simulink model "junyakaiguangai5"  (Simulink 8.8)
settings: Solver=ode4  StartTime=0.0  StopTime=inf  FixedStep=0.001  RelTol=1e-3  EnableMultiTasking=on
undefined symbols (not defined in the file or in its folder): mdaadlink6208, sigbuilder_block
libraries: xpcobsoletelib x24, slrtlib x2, simulink x1
(part 2 of 3)

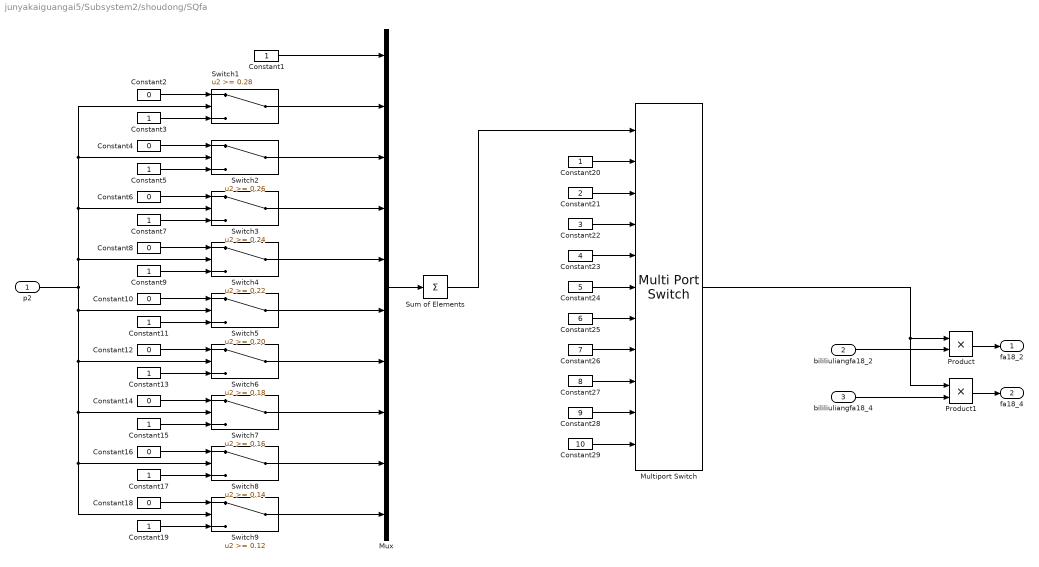
== system junyakaiguangai5/Subsystem2/shoudong/SQfa ==
  p2 : Inport
  bililiuliangfa18_2 : Inport  Port=2
  bililiuliangfa18_4 : Inport  Port=3
  Constant{1,3,5,7,9,11,13,15,17,19..20} (11 alike) : Constant
  Constant{2,4,6,8,10,12,14,16,18} (9 alike) : Constant  Value=0
  Constant21 : Constant  Value=2
  Constant22 : Constant  Value=3
  Constant23 : Constant  Value=4
  Constant24 : Constant  Value=5
  Constant25 : Constant  Value=6
  Constant26 : Constant  Value=7
  Constant27 : Constant  Value=8
  Constant28 : Constant  Value=9
  Constant29 : Constant  Value=10
  Multiport Switch : MultiPortSwitch  Inputs=10
  Mux : Mux  Inputs=10
  Product : Product  RndMeth=Zero
  Product1 : Product  RndMeth=Zero
  Sum of Elements : Sum  Inputs=+
  Switch1 : Switch  Threshold=0.28
  Switch2 : Switch  Threshold=0.26
  Switch3 : Switch  Threshold=0.24
  Switch4 : Switch  Threshold=0.22
  Switch5 : Switch  Threshold=0.20
  Switch6 : Switch  Threshold=0.18
  Switch7 : Switch  Threshold=0.16
  Switch8 : Switch  Threshold=0.14
  Switch9 : Switch  Threshold=0.12
  fa18_2 : Outport
  fa18_4 : Outport  Port=2
  wires:
  Constant2/1 -> Switch1/1
  Constant3/1 -> Switch1/3
  Constant4/1 -> Switch2/1
  Constant5/1 -> Switch2/3
  Constant6/1 -> Switch3/1
  Constant7/1 -> Switch3/3
  Constant8/1 -> Switch4/1
  Constant9/1 -> Switch4/3
  Constant10/1 -> Switch5/1
  Constant11/1 -> Switch5/3
  Constant12/1 -> Switch6/1
  Constant13/1 -> Switch6/3
  Constant14/1 -> Switch7/1
  Constant15/1 -> Switch7/3
  p2/1 -> Switch1/2, Switch2/2, Switch3/2, Switch4/2, Switch6/2, Switch7/2, Switch8/2, Switch9/2, Switch5/2
  Mux/1 -> Sum of Elements/1
  Sum of Elements/1 -> Multiport Switch/1
  Constant1/1 -> Mux/1
  Switch1/1 -> Mux/2
  Switch2/1 -> Mux/3
  Switch3/1 -> Mux/4
  Switch4/1 -> Mux/5
  Switch5/1 -> Mux/6
  Switch6/1 -> Mux/7
  Switch7/1 -> Mux/8
  Switch8/1 -> Mux/9
  Switch9/1 -> Mux/10
  Constant16/1 -> Switch8/1
  Constant17/1 -> Switch8/3
  Constant18/1 -> Switch9/1
  Constant19/1 -> Switch9/3
  Multiport Switch/1 -> Product/1, Product1/1
  Constant20/1 -> Multiport Switch/2
  Constant21/1 -> Multiport Switch/3
  Constant22/1 -> Multiport Switch/4
  Constant23/1 -> Multiport Switch/5
  Constant24/1 -> Multiport Switch/6
  Constant25/1 -> Multiport Switch/7
  Constant26/1 -> Multiport Switch/8
  Constant27/1 -> Multiport Switch/9
  Constant28/1 -> Multiport Switch/10
  Constant29/1 -> Multiport Switch/11
  bililiuliangfa18_2/1 -> Product/2
  bililiuliangfa18_4/1 -> Product1/2
  Product/1 -> fa18_2/1
  Product1/1 -> fa18_4/1

== system junyakaiguangai5/Subsystem2/shoudong/Subsystem1 ==
  kaigaikaishi : Inport
  guangaikaishi : Inport  Port=2
  xkgg : Inport  Port=3
  Add1 : Sum
  Constant : Constant  Value=2
  Constant1 : Constant  Value=0
  Gain : Gain
  Gain1 : Gain
  Multiport Switch : MultiPortSwitch
  Product : Product
  Signal Builder : Subsystem  Tag=STV Subsys  LoadFcn=sigbuilder_block('load');  StartFcn=sigbuilder_block('start');  StopFcn=sigbuilder_block('stop');  ClipboardFcn=sigbuilder_block('clipboard');  mask(Sigbuilder block){tuvar=[0:10]}
      mask help: Simulink:masks:SigbuilderBlock_MD
      mask init:
      | if ~strcmp(get_param(bdroot(gcbh),'SimulationStatus'),'stopped') tuvar = sigbuilder_block('maskInit'); end
      settings: CopyFcn=sigbuilder_block('copy');  DeleteFcn=sigbuilder_block('delete');  ModelCloseFcn=sigbuilder_block('modelClose');  PreSaveFcn=sigbuilder_block('preSave');  PauseFcn=sigbuilder_block('pause');  ContinueFcn=sigbuilder_block('continue');  NameChangeFcn=sigbuilder_block('namechange');  OpenFcn=sigbuilder_block('open',[437.6 199.2 550.4 400 ]);  CloseFcn=sigbuilder_block('close');
      mask Display: plot(0, 0, 100, 100,[2, 2, 32, 32, 2], [68, 8, 8, 68, 68],[32, 2], [38, 38], [32, 19, 2],[53, 60, 44], [32, 17, 17, 2],[16, 16, 31, 31]);txt = getActiveGroup(gcbh);text(2, 100, txt,'verticalAlignment', 'top');
  Signal Builder1 : Subsystem  Tag=STV Subsys  LoadFcn=sigbuilder_block('load');  StartFcn=sigbuilder_block('start');  StopFcn=sigbuilder_block('stop');  ClipboardFcn=sigbuilder_block('clipboard');  mask(Sigbuilder block){tuvar=[0:10]}
      mask help: Simulink:masks:SigbuilderBlock_MD
      mask init:
      | if ~strcmp(get_param(bdroot(gcbh),'SimulationStatus'),'stopped') tuvar = sigbuilder_block('maskInit'); end
      settings: CopyFcn=sigbuilder_block('copy');  DeleteFcn=sigbuilder_block('delete');  ModelCloseFcn=sigbuilder_block('modelClose');  PreSaveFcn=sigbuilder_block('preSave');  PauseFcn=sigbuilder_block('pause');  ContinueFcn=sigbuilder_block('continue');  NameChangeFcn=sigbuilder_block('namechange');  OpenFcn=sigbuilder_block('open',[437.6 199.2 550.4 400 ]);  CloseFcn=sigbuilder_block('close');
      mask Display: plot(0, 0, 100, 100,[2, 2, 32, 32, 2], [68, 8, 8, 68, 68],[32, 2], [38, 38], [32, 19, 2],[53, 60, 44], [32, 17, 17, 2],[16, 16, 31, 31]);txt = getActiveGroup(gcbh);text(2, 100, txt,'verticalAlignment', 'top');
  Sum : Sum  Inputs=|+-
  Sum1 : Sum  Inputs=|+-
  Out1 : Outport
  wires:
  guangaikaishi/1 -> Product/1
  Constant/1 -> Product/2
  kaigaikaishi/1 -> Add1/1
  Product/1 -> Add1/2
  Add1/1 -> Multiport Switch/1
  Multiport Switch/1 -> Out1/1
  Signal Builder/1(Signal 1) -> Sum/1
  xkgg/1 -> Sum1/2, Sum/2
  Sum/1 -> Gain/1
  Gain/1 -> Multiport Switch/2
  Signal Builder1/1(Signal 1) -> Sum1/1
  Sum1/1 -> Gain1/1
  Gain1/1 -> Multiport Switch/3
  Constant1/1 -> Multiport Switch/4

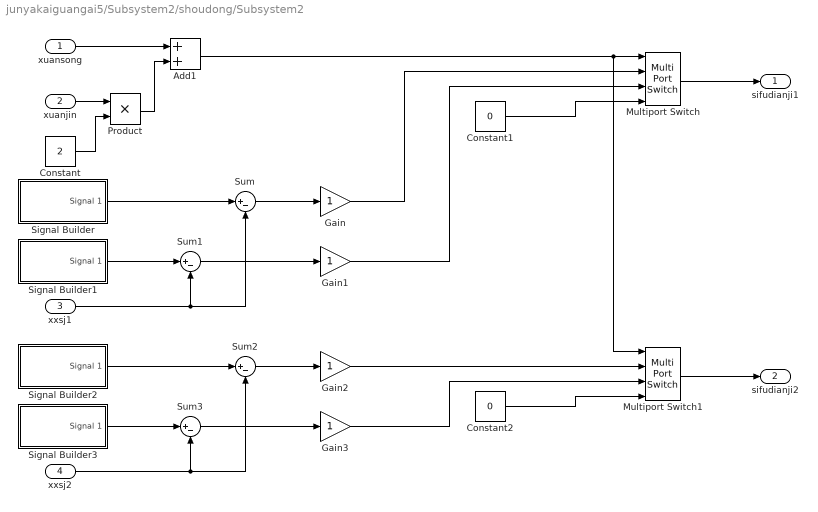
== system junyakaiguangai5/Subsystem2/shoudong/Subsystem2 ==
  xuansong : Inport
  xuanjin : Inport  Port=2
  xxsj1 : Inport  Port=3
  xxsj2 : Inport  Port=4
  Add1 : Sum
  Constant : Constant  Value=2
  Constant1 : Constant  Value=0
  Constant2 : Constant  Value=0
  Gain{,1..3} (4 alike) : Gain
  Multiport Switch : MultiPortSwitch
  Multiport Switch1 : MultiPortSwitch
  Product : Product
  Signal Builder : Subsystem  Tag=STV Subsys  LoadFcn=sigbuilder_block('load');  StartFcn=sigbuilder_block('start');  StopFcn=sigbuilder_block('stop');  ClipboardFcn=sigbuilder_block('clipboard');  mask(Sigbuilder block){tuvar=[0:10]}
      mask help: Simulink:masks:SigbuilderBlock_MD
      mask init:
      | if ~strcmp(get_param(bdroot(gcbh),'SimulationStatus'),'stopped') tuvar = sigbuilder_block('maskInit'); end
      settings: CopyFcn=sigbuilder_block('copy');  DeleteFcn=sigbuilder_block('delete');  ModelCloseFcn=sigbuilder_block('modelClose');  PreSaveFcn=sigbuilder_block('preSave');  PauseFcn=sigbuilder_block('pause');  ContinueFcn=sigbuilder_block('continue');  NameChangeFcn=sigbuilder_block('namechange');  OpenFcn=sigbuilder_block('open',[437.6 199.2 550.4 400 ]);  CloseFcn=sigbuilder_block('close');
      mask Display: plot(0, 0, 100, 100,[2, 2, 32, 32, 2], [68, 8, 8, 68, 68],[32, 2], [38, 38], [32, 19, 2],[53, 60, 44], [32, 17, 17, 2],[16, 16, 31, 31]);txt = getActiveGroup(gcbh);text(2, 100, txt,'verticalAlignment', 'top');
  Signal Builder1 : Subsystem  Tag=STV Subsys  LoadFcn=sigbuilder_block('load');  StartFcn=sigbuilder_block('start');  StopFcn=sigbuilder_block('stop');  ClipboardFcn=sigbuilder_block('clipboard');  mask(Sigbuilder block){tuvar=[0:10]}
      mask help: Simulink:masks:SigbuilderBlock_MD
      mask init:
      | if ~strcmp(get_param(bdroot(gcbh),'SimulationStatus'),'stopped') tuvar = sigbuilder_block('maskInit'); end
      settings: CopyFcn=sigbuilder_block('copy');  DeleteFcn=sigbuilder_block('delete');  ModelCloseFcn=sigbuilder_block('modelClose');  PreSaveFcn=sigbuilder_block('preSave');  PauseFcn=sigbuilder_block('pause');  ContinueFcn=sigbuilder_block('continue');  NameChangeFcn=sigbuilder_block('namechange');  OpenFcn=sigbuilder_block('open',[437.6 199.2 550.4 400 ]);  CloseFcn=sigbuilder_block('close');
      mask Display: plot(0, 0, 100, 100,[2, 2, 32, 32, 2], [68, 8, 8, 68, 68],[32, 2], [38, 38], [32, 19, 2],[53, 60, 44], [32, 17, 17, 2],[16, 16, 31, 31]);txt = getActiveGroup(gcbh);text(2, 100, txt,'verticalAlignment', 'top');
  Signal Builder2 : Subsystem  Tag=STV Subsys  LoadFcn=sigbuilder_block('load');  StartFcn=sigbuilder_block('start');  StopFcn=sigbuilder_block('stop');  ClipboardFcn=sigbuilder_block('clipboard');  mask(Sigbuilder block){tuvar=[0:10]}
      mask help: Simulink:masks:SigbuilderBlock_MD
      mask init:
      | if ~strcmp(get_param(bdroot(gcbh),'SimulationStatus'),'stopped') tuvar = sigbuilder_block('maskInit'); end
      settings: CopyFcn=sigbuilder_block('copy');  DeleteFcn=sigbuilder_block('delete');  ModelCloseFcn=sigbuilder_block('modelClose');  PreSaveFcn=sigbuilder_block('preSave');  PauseFcn=sigbuilder_block('pause');  ContinueFcn=sigbuilder_block('continue');  NameChangeFcn=sigbuilder_block('namechange');  OpenFcn=sigbuilder_block('open',[437.6 199.2 550.4 400 ]);  CloseFcn=sigbuilder_block('close');
      mask Display: plot(0, 0, 100, 100,[2, 2, 32, 32, 2], [68, 8, 8, 68, 68],[32, 2], [38, 38], [32, 19, 2],[53, 60, 44], [32, 17, 17, 2],[16, 16, 31, 31]);txt = getActiveGroup(gcbh);text(2, 100, txt,'verticalAlignment', 'top');
  Signal Builder3 : Subsystem  Tag=STV Subsys  LoadFcn=sigbuilder_block('load');  StartFcn=sigbuilder_block('start');  StopFcn=sigbuilder_block('stop');  ClipboardFcn=sigbuilder_block('clipboard');  mask(Sigbuilder block){tuvar=[0:10]}
      mask help: Simulink:masks:SigbuilderBlock_MD
      mask init:
      | if ~strcmp(get_param(bdroot(gcbh),'SimulationStatus'),'stopped') tuvar = sigbuilder_block('maskInit'); end
      settings: CopyFcn=sigbuilder_block('copy');  DeleteFcn=sigbuilder_block('delete');  ModelCloseFcn=sigbuilder_block('modelClose');  PreSaveFcn=sigbuilder_block('preSave');  PauseFcn=sigbuilder_block('pause');  ContinueFcn=sigbuilder_block('continue');  NameChangeFcn=sigbuilder_block('namechange');  OpenFcn=sigbuilder_block('open',[437.6 199.2 550.4 400 ]);  CloseFcn=sigbuilder_block('close');
      mask Display: plot(0, 0, 100, 100,[2, 2, 32, 32, 2], [68, 8, 8, 68, 68],[32, 2], [38, 38], [32, 19, 2],[53, 60, 44], [32, 17, 17, 2],[16, 16, 31, 31]);txt = getActiveGroup(gcbh);text(2, 100, txt,'verticalAlignment', 'top');
  Sum{,1..3} (4 alike) : Sum  Inputs=|+-
  sifudianji1 : Outport
  sifudianji2 : Outport  Port=2
  wires:
  Constant1/1 -> Multiport Switch/4
  Gain1/1 -> Multiport Switch/3
  Sum1/1 -> Gain1/1
  Signal Builder1/1(Signal 1) -> Sum1/1
  Gain/1 -> Multiport Switch/2
  Sum/1 -> Gain/1
  xxsj1/1 -> Sum/2, Sum1/2
  Signal Builder/1(Signal 1) -> Sum/1
  Multiport Switch/1 -> sifudianji1/1
  Add1/1 -> Multiport Switch1/1, Multiport Switch/1
  Product/1 -> Add1/2
  xuansong/1 -> Add1/1
  Constant/1 -> Product/2
  xuanjin/1 -> Product/1
  Multiport Switch1/1 -> sifudianji2/1
  Signal Builder2/1(Signal 1) -> Sum2/1
  xxsj2/1 -> Sum2/2, Sum3/2
  Sum2/1 -> Gain2/1
  Gain2/1 -> Multiport Switch1/2
  Signal Builder3/1(Signal 1) -> Sum3/1
  Sum3/1 -> Gain3/1
  Gain3/1 -> Multiport Switch1/3
  Constant2/1 -> Multiport Switch1/4

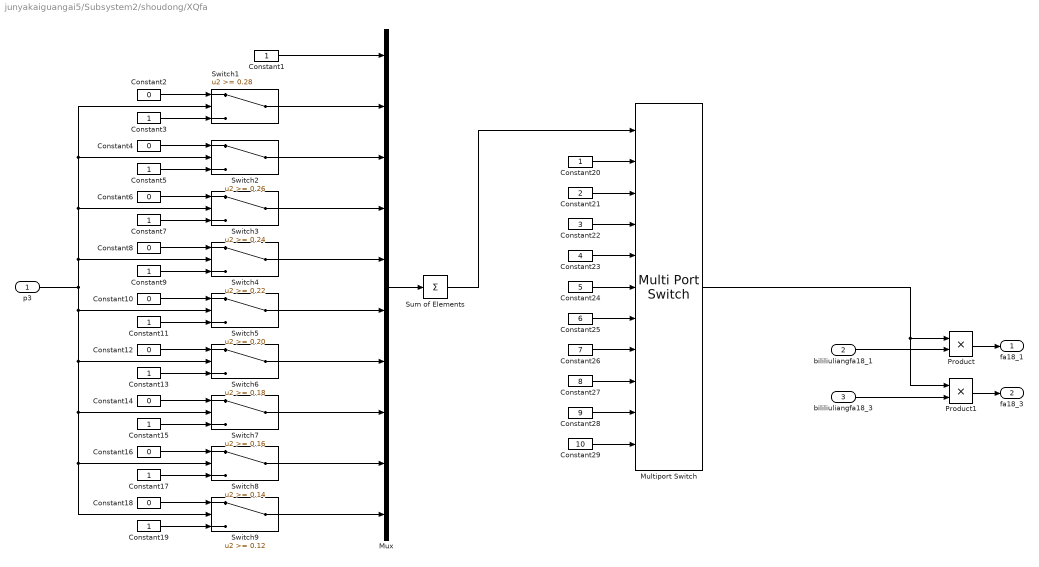
== system junyakaiguangai5/Subsystem2/shoudong/XQfa ==
  p3 : Inport
  bililiuliangfa18_1 : Inport  Port=2
  bililiuliangfa18_3 : Inport  Port=3
  Constant{1,3,5,7,9,11,13,15,17,19..20} (11 alike) : Constant
  Constant{2,4,6,8,10,12,14,16,18} (9 alike) : Constant  Value=0
  Constant21 : Constant  Value=2
  Constant22 : Constant  Value=3
  Constant23 : Constant  Value=4
  Constant24 : Constant  Value=5
  Constant25 : Constant  Value=6
  Constant26 : Constant  Value=7
  Constant27 : Constant  Value=8
  Constant28 : Constant  Value=9
  Constant29 : Constant  Value=10
  Multiport Switch : MultiPortSwitch  Inputs=10
  Mux : Mux  Inputs=10
  Product : Product  RndMeth=Zero
  Product1 : Product  RndMeth=Zero
  Sum of Elements : Sum  Inputs=+
  Switch1 : Switch  Threshold=0.28
  Switch2 : Switch  Threshold=0.26
  Switch3 : Switch  Threshold=0.24
  Switch4 : Switch  Threshold=0.22
  Switch5 : Switch  Threshold=0.20
  Switch6 : Switch  Threshold=0.18
  Switch7 : Switch  Threshold=0.16
  Switch8 : Switch  Threshold=0.14
  Switch9 : Switch  Threshold=0.12
  fa18_1 : Outport
  fa18_3 : Outport  Port=2
  wires:
  Product1/1 -> fa18_3/1
  Product/1 -> fa18_1/1
  bililiuliangfa18_3/1 -> Product1/2
  bililiuliangfa18_1/1 -> Product/2
  Constant29/1 -> Multiport Switch/11
  Constant28/1 -> Multiport Switch/10
  Constant27/1 -> Multiport Switch/9
  Constant26/1 -> Multiport Switch/8
  Constant25/1 -> Multiport Switch/7
  Constant24/1 -> Multiport Switch/6
  Constant23/1 -> Multiport Switch/5
  Constant22/1 -> Multiport Switch/4
  Constant21/1 -> Multiport Switch/3
  Constant20/1 -> Multiport Switch/2
  Multiport Switch/1 -> Product1/1, Product/1
  Constant19/1 -> Switch9/3
  Constant18/1 -> Switch9/1
  Constant17/1 -> Switch8/3
  Constant16/1 -> Switch8/1
  Switch9/1 -> Mux/10
  Switch8/1 -> Mux/9
  Switch7/1 -> Mux/8
  Switch6/1 -> Mux/7
  Switch5/1 -> Mux/6
  Switch4/1 -> Mux/5
  Switch3/1 -> Mux/4
  Switch2/1 -> Mux/3
  Switch1/1 -> Mux/2
  Constant1/1 -> Mux/1
  Sum of Elements/1 -> Multiport Switch/1
  Mux/1 -> Sum of Elements/1
  p3/1 -> Switch5/2, Switch9/2, Switch8/2, Switch7/2, Switch6/2, Switch4/2, Switch3/2, Switch2/2, Switch1/2
  Constant15/1 -> Switch7/3
  Constant14/1 -> Switch7/1
  Constant13/1 -> Switch6/3
  Constant12/1 -> Switch6/1
  Constant11/1 -> Switch5/3
  Constant10/1 -> Switch5/1
  Constant9/1 -> Switch4/3
  Constant8/1 -> Switch4/1
  Constant7/1 -> Switch3/3
  Constant6/1 -> Switch3/1
  Constant5/1 -> Switch2/3
  Constant4/1 -> Switch2/1
  Constant3/1 -> Switch1/3
  Constant2/1 -> Switch1/1

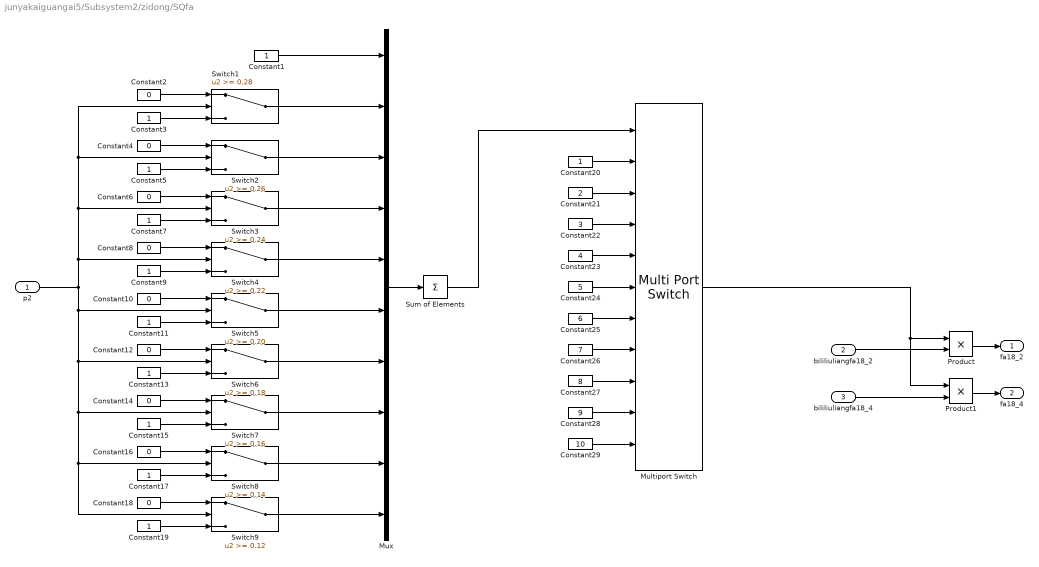
== system junyakaiguangai5/Subsystem2/zidong/SQfa ==
  p2 : Inport
  bililiuliangfa18_2 : Inport  Port=2
  bililiuliangfa18_4 : Inport  Port=3
  Constant{1,3,5,7,9,11,13,15,17,19..20} (11 alike) : Constant
  Constant{2,4,6,8,10,12,14,16,18} (9 alike) : Constant  Value=0
  Constant21 : Constant  Value=2
  Constant22 : Constant  Value=3
  Constant23 : Constant  Value=4
  Constant24 : Constant  Value=5
  Constant25 : Constant  Value=6
  Constant26 : Constant  Value=7
  Constant27 : Constant  Value=8
  Constant28 : Constant  Value=9
  Constant29 : Constant  Value=10
  Multiport Switch : MultiPortSwitch  Inputs=10
  Mux : Mux  Inputs=10
  Product : Product  RndMeth=Zero
  Product1 : Product  RndMeth=Zero
  Sum of Elements : Sum  Inputs=+
  Switch1 : Switch  Threshold=0.28
  Switch2 : Switch  Threshold=0.26
  Switch3 : Switch  Threshold=0.24
  Switch4 : Switch  Threshold=0.22
  Switch5 : Switch  Threshold=0.20
  Switch6 : Switch  Threshold=0.18
  Switch7 : Switch  Threshold=0.16
  Switch8 : Switch  Threshold=0.14
  Switch9 : Switch  Threshold=0.12
  fa18_2 : Outport
  fa18_4 : Outport  Port=2
  wires:
  Product1/1 -> fa18_4/1
  Product/1 -> fa18_2/1
  bililiuliangfa18_4/1 -> Product1/2
  bililiuliangfa18_2/1 -> Product/2
  Constant29/1 -> Multiport Switch/11
  Constant28/1 -> Multiport Switch/10
  Constant27/1 -> Multiport Switch/9
  Constant26/1 -> Multiport Switch/8
  Constant25/1 -> Multiport Switch/7
  Constant24/1 -> Multiport Switch/6
  Constant23/1 -> Multiport Switch/5
  Constant22/1 -> Multiport Switch/4
  Constant21/1 -> Multiport Switch/3
  Constant20/1 -> Multiport Switch/2
  Multiport Switch/1 -> Product1/1, Product/1
  Constant19/1 -> Switch9/3
  Constant18/1 -> Switch9/1
  Constant17/1 -> Switch8/3
  Constant16/1 -> Switch8/1
  Switch9/1 -> Mux/10
  Switch8/1 -> Mux/9
  Switch7/1 -> Mux/8
  Switch6/1 -> Mux/7
  Switch5/1 -> Mux/6
  Switch4/1 -> Mux/5
  Switch3/1 -> Mux/4
  Switch2/1 -> Mux/3
  Switch1/1 -> Mux/2
  Constant1/1 -> Mux/1
  Sum of Elements/1 -> Multiport Switch/1
  Mux/1 -> Sum of Elements/1
  p2/1 -> Switch5/2, Switch9/2, Switch8/2, Switch7/2, Switch6/2, Switch4/2, Switch3/2, Switch2/2, Switch1/2
  Constant15/1 -> Switch7/3
  Constant14/1 -> Switch7/1
  Constant13/1 -> Switch6/3
  Constant12/1 -> Switch6/1
  Constant11/1 -> Switch5/3
  Constant10/1 -> Switch5/1
  Constant9/1 -> Switch4/3
  Constant8/1 -> Switch4/1
  Constant7/1 -> Switch3/3
  Constant6/1 -> Switch3/1
  Constant5/1 -> Switch2/3
  Constant4/1 -> Switch2/1
  Constant3/1 -> Switch1/3
  Constant2/1 -> Switch1/1

== system junyakaiguangai5/Subsystem2/zidong/Subsystem ==
  kaigaikaishi : Inport
  guangaikaishi : Inport  Port=2
  xkgg : Inport  Port=3
  Add1 : Sum
  Constant : Constant  Value=2
  Constant1 : Constant  Value=0
  Gain : Gain
  Gain1 : Gain
  Multiport Switch : MultiPortSwitch
  Product : Product
  Signal Builder : Subsystem  Tag=STV Subsys  LoadFcn=sigbuilder_block('load');  StartFcn=sigbuilder_block('start');  StopFcn=sigbuilder_block('stop');  ClipboardFcn=sigbuilder_block('clipboard');  mask(Sigbuilder block){tuvar=[0:10]}
      mask help: Simulink:masks:SigbuilderBlock_MD
      mask init:
      | if ~strcmp(get_param(bdroot(gcbh),'SimulationStatus'),'stopped') tuvar = sigbuilder_block('maskInit'); end
      settings: CopyFcn=sigbuilder_block('copy');  DeleteFcn=sigbuilder_block('delete');  ModelCloseFcn=sigbuilder_block('modelClose');  PreSaveFcn=sigbuilder_block('preSave');  PauseFcn=sigbuilder_block('pause');  ContinueFcn=sigbuilder_block('continue');  NameChangeFcn=sigbuilder_block('namechange');  OpenFcn=sigbuilder_block('open',[440.25 156.75 544.5 354.75 ]);  CloseFcn=sigbuilder_block('close');
      mask Display: plot(0, 0, 100, 100,[2, 2, 32, 32, 2], [68, 8, 8, 68, 68],[32, 2], [38, 38], [32, 19, 2],[53, 60, 44], [32, 17, 17, 2],[16, 16, 31, 31]);txt = getActiveGroup(gcbh);text(2, 100, txt,'verticalAlignment', 'top');
  Signal Builder1 : Subsystem  Tag=STV Subsys  LoadFcn=sigbuilder_block('load');  StartFcn=sigbuilder_block('start');  StopFcn=sigbuilder_block('stop');  ClipboardFcn=sigbuilder_block('clipboard');  mask(Sigbuilder block){tuvar=[0:10]}
      mask help: Simulink:masks:SigbuilderBlock_MD
      mask init:
      | if ~strcmp(get_param(bdroot(gcbh),'SimulationStatus'),'stopped') tuvar = sigbuilder_block('maskInit'); end
      settings: CopyFcn=sigbuilder_block('copy');  DeleteFcn=sigbuilder_block('delete');  ModelCloseFcn=sigbuilder_block('modelClose');  PreSaveFcn=sigbuilder_block('preSave');  PauseFcn=sigbuilder_block('pause');  ContinueFcn=sigbuilder_block('continue');  NameChangeFcn=sigbuilder_block('namechange');  OpenFcn=sigbuilder_block('open',[437.6 199.2 550.4 400 ]);  CloseFcn=sigbuilder_block('close');
      mask Display: plot(0, 0, 100, 100,[2, 2, 32, 32, 2], [68, 8, 8, 68, 68],[32, 2], [38, 38], [32, 19, 2],[53, 60, 44], [32, 17, 17, 2],[16, 16, 31, 31]);txt = getActiveGroup(gcbh);text(2, 100, txt,'verticalAlignment', 'top');
  Sum : Sum  Inputs=|+-
  Sum1 : Sum  Inputs=|+-
  Out1 : Outport
  wires:
  guangaikaishi/1 -> Product/1
  Constant/1 -> Product/2
  kaigaikaishi/1 -> Add1/1
  Product/1 -> Add1/2
  Add1/1 -> Multiport Switch/1
  Multiport Switch/1 -> Out1/1
  Signal Builder/1(Signal 1) -> Sum/1
  xkgg/1 -> Sum1/2, Sum/2
  Sum/1 -> Gain/1
  Gain/1 -> Multiport Switch/2
  Signal Builder1/1(Signal 1) -> Sum1/1
  Sum1/1 -> Gain1/1
  Gain1/1 -> Multiport Switch/3
  Constant1/1 -> Multiport Switch/4

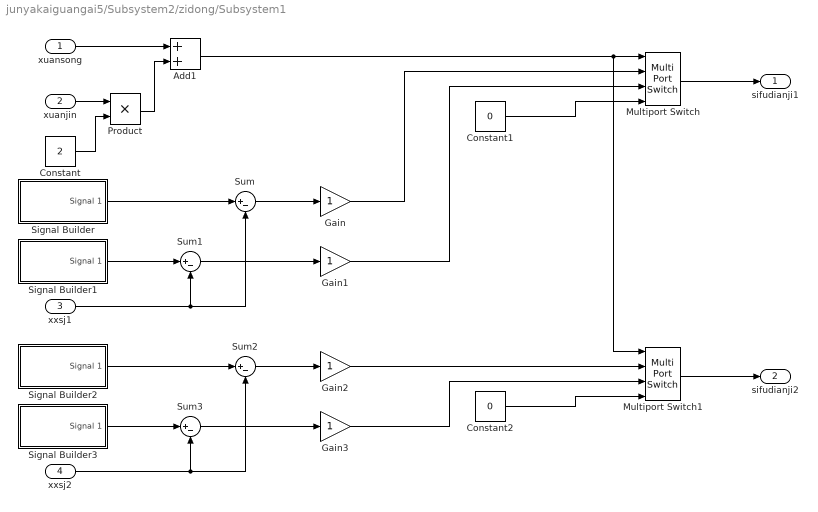
== system junyakaiguangai5/Subsystem2/zidong/Subsystem1 ==
  xuansong : Inport
  xuanjin : Inport  Port=2
  xxsj1 : Inport  Port=3
  xxsj2 : Inport  Port=4
  Add1 : Sum
  Constant : Constant  Value=2
  Constant1 : Constant  Value=0
  Constant2 : Constant  Value=0
  Gain{,1..3} (4 alike) : Gain
  Multiport Switch : MultiPortSwitch
  Multiport Switch1 : MultiPortSwitch
  Product : Product
  Signal Builder : Subsystem  Tag=STV Subsys  LoadFcn=sigbuilder_block('load');  StartFcn=sigbuilder_block('start');  StopFcn=sigbuilder_block('stop');  ClipboardFcn=sigbuilder_block('clipboard');  mask(Sigbuilder block){tuvar=[0:10]}
      mask help: Simulink:masks:SigbuilderBlock_MD
      mask init:
      | if ~strcmp(get_param(bdroot(gcbh),'SimulationStatus'),'stopped') tuvar = sigbuilder_block('maskInit'); end
      settings: CopyFcn=sigbuilder_block('copy');  DeleteFcn=sigbuilder_block('delete');  ModelCloseFcn=sigbuilder_block('modelClose');  PreSaveFcn=sigbuilder_block('preSave');  PauseFcn=sigbuilder_block('pause');  ContinueFcn=sigbuilder_block('continue');  NameChangeFcn=sigbuilder_block('namechange');  OpenFcn=sigbuilder_block('open',[437.6 199.2 550.4 400 ]);  CloseFcn=sigbuilder_block('close');
      mask Display: plot(0, 0, 100, 100,[2, 2, 32, 32, 2], [68, 8, 8, 68, 68],[32, 2], [38, 38], [32, 19, 2],[53, 60, 44], [32, 17, 17, 2],[16, 16, 31, 31]);txt = getActiveGroup(gcbh);text(2, 100, txt,'verticalAlignment', 'top');
  Signal Builder1 : Subsystem  Tag=STV Subsys  LoadFcn=sigbuilder_block('load');  StartFcn=sigbuilder_block('start');  StopFcn=sigbuilder_block('stop');  ClipboardFcn=sigbuilder_block('clipboard');  mask(Sigbuilder block){tuvar=[0:10]}
      mask help: Simulink:masks:SigbuilderBlock_MD
      mask init:
      | if ~strcmp(get_param(bdroot(gcbh),'SimulationStatus'),'stopped') tuvar = sigbuilder_block('maskInit'); end
      settings: CopyFcn=sigbuilder_block('copy');  DeleteFcn=sigbuilder_block('delete');  ModelCloseFcn=sigbuilder_block('modelClose');  PreSaveFcn=sigbuilder_block('preSave');  PauseFcn=sigbuilder_block('pause');  ContinueFcn=sigbuilder_block('continue');  NameChangeFcn=sigbuilder_block('namechange');  OpenFcn=sigbuilder_block('open',[437.6 199.2 550.4 400 ]);  CloseFcn=sigbuilder_block('close');
      mask Display: plot(0, 0, 100, 100,[2, 2, 32, 32, 2], [68, 8, 8, 68, 68],[32, 2], [38, 38], [32, 19, 2],[53, 60, 44], [32, 17, 17, 2],[16, 16, 31, 31]);txt = getActiveGroup(gcbh);text(2, 100, txt,'verticalAlignment', 'top');
  Signal Builder2 : Subsystem  Tag=STV Subsys  LoadFcn=sigbuilder_block('load');  StartFcn=sigbuilder_block('start');  StopFcn=sigbuilder_block('stop');  ClipboardFcn=sigbuilder_block('clipboard');  mask(Sigbuilder block){tuvar=[0:10]}
      mask help: Simulink:masks:SigbuilderBlock_MD
      mask init:
      | if ~strcmp(get_param(bdroot(gcbh),'SimulationStatus'),'stopped') tuvar = sigbuilder_block('maskInit'); end
      settings: CopyFcn=sigbuilder_block('copy');  DeleteFcn=sigbuilder_block('delete');  ModelCloseFcn=sigbuilder_block('modelClose');  PreSaveFcn=sigbuilder_block('preSave');  PauseFcn=sigbuilder_block('pause');  ContinueFcn=sigbuilder_block('continue');  NameChangeFcn=sigbuilder_block('namechange');  OpenFcn=sigbuilder_block('open',[437.6 199.2 550.4 400 ]);  CloseFcn=sigbuilder_block('close');
      mask Display: plot(0, 0, 100, 100,[2, 2, 32, 32, 2], [68, 8, 8, 68, 68],[32, 2], [38, 38], [32, 19, 2],[53, 60, 44], [32, 17, 17, 2],[16, 16, 31, 31]);txt = getActiveGroup(gcbh);text(2, 100, txt,'verticalAlignment', 'top');
  Signal Builder3 : Subsystem  Tag=STV Subsys  LoadFcn=sigbuilder_block('load');  StartFcn=sigbuilder_block('start');  StopFcn=sigbuilder_block('stop');  ClipboardFcn=sigbuilder_block('clipboard');  mask(Sigbuilder block){tuvar=[0:10]}
      mask help: Simulink:masks:SigbuilderBlock_MD
      mask init:
      | if ~strcmp(get_param(bdroot(gcbh),'SimulationStatus'),'stopped') tuvar = sigbuilder_block('maskInit'); end
      settings: CopyFcn=sigbuilder_block('copy');  DeleteFcn=sigbuilder_block('delete');  ModelCloseFcn=sigbuilder_block('modelClose');  PreSaveFcn=sigbuilder_block('preSave');  PauseFcn=sigbuilder_block('pause');  ContinueFcn=sigbuilder_block('continue');  NameChangeFcn=sigbuilder_block('namechange');  OpenFcn=sigbuilder_block('open',[437.6 199.2 550.4 400 ]);  CloseFcn=sigbuilder_block('close');
      mask Display: plot(0, 0, 100, 100,[2, 2, 32, 32, 2], [68, 8, 8, 68, 68],[32, 2], [38, 38], [32, 19, 2],[53, 60, 44], [32, 17, 17, 2],[16, 16, 31, 31]);txt = getActiveGroup(gcbh);text(2, 100, txt,'verticalAlignment', 'top');
  Sum{,1..3} (4 alike) : Sum  Inputs=|+-
  sifudianji1 : Outport
  sifudianji2 : Outport  Port=2
  wires:
  Constant1/1 -> Multiport Switch/4
  Gain1/1 -> Multiport Switch/3
  Sum1/1 -> Gain1/1
  Signal Builder1/1(Signal 1) -> Sum1/1
  Gain/1 -> Multiport Switch/2
  Sum/1 -> Gain/1
  xxsj1/1 -> Sum/2, Sum1/2
  Signal Builder/1(Signal 1) -> Sum/1
  Multiport Switch/1 -> sifudianji1/1
  Add1/1 -> Multiport Switch1/1, Multiport Switch/1
  Product/1 -> Add1/2
  xuansong/1 -> Add1/1
  Constant/1 -> Product/2
  xuanjin/1 -> Product/1
  Multiport Switch1/1 -> sifudianji2/1
  Signal Builder2/1(Signal 1) -> Sum2/1
  xxsj2/1 -> Sum2/2, Sum3/2
  Sum2/1 -> Gain2/1
  Gain2/1 -> Multiport Switch1/2
  Signal Builder3/1(Signal 1) -> Sum3/1
  Sum3/1 -> Gain3/1
  Gain3/1 -> Multiport Switch1/3
  Constant2/1 -> Multiport Switch1/4

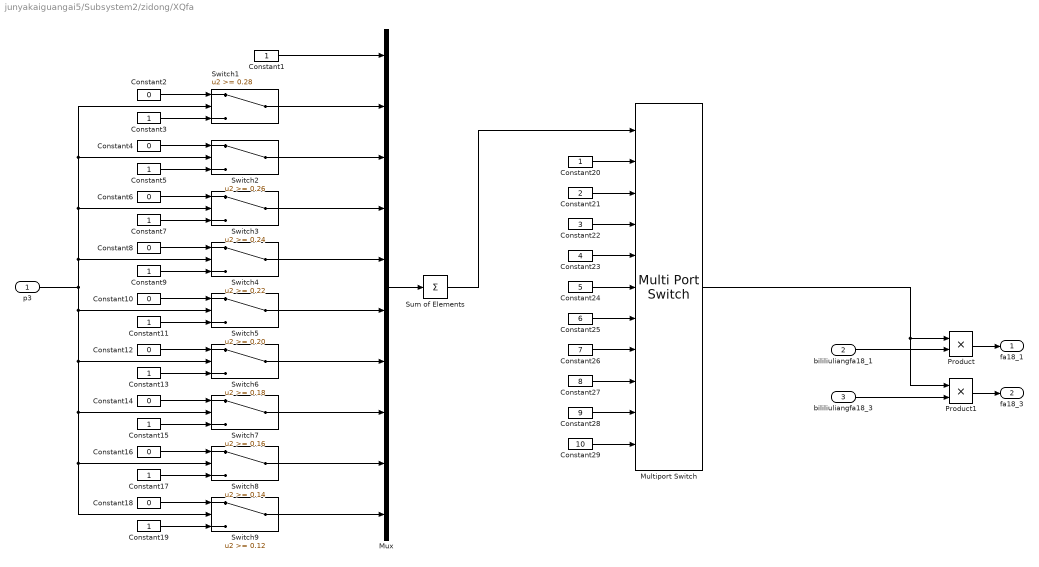
== system junyakaiguangai5/Subsystem2/zidong/XQfa ==
  p3 : Inport
  bililiuliangfa18_1 : Inport  Port=2
  bililiuliangfa18_3 : Inport  Port=3
  Constant{1,3,5,7,9,11,13,15,17,19..20} (11 alike) : Constant
  Constant{2,4,6,8,10,12,14,16,18} (9 alike) : Constant  Value=0
  Constant21 : Constant  Value=2
  Constant22 : Constant  Value=3
  Constant23 : Constant  Value=4
  Constant24 : Constant  Value=5
  Constant25 : Constant  Value=6
  Constant26 : Constant  Value=7
  Constant27 : Constant  Value=8
  Constant28 : Constant  Value=9
  Constant29 : Constant  Value=10
  Multiport Switch : MultiPortSwitch  Inputs=10
  Mux : Mux  Inputs=10
  Product : Product  RndMeth=Zero
  Product1 : Product  RndMeth=Zero
  Sum of Elements : Sum  Inputs=+
  Switch1 : Switch  Threshold=0.28
  Switch2 : Switch  Threshold=0.26
  Switch3 : Switch  Threshold=0.24
  Switch4 : Switch  Threshold=0.22
  Switch5 : Switch  Threshold=0.20
  Switch6 : Switch  Threshold=0.18
  Switch7 : Switch  Threshold=0.16
  Switch8 : Switch  Threshold=0.14
  Switch9 : Switch  Threshold=0.12
  fa18_1 : Outport
  fa18_3 : Outport  Port=2
  wires:
  Constant2/1 -> Switch1/1
  Constant3/1 -> Switch1/3
  Constant4/1 -> Switch2/1
  Constant5/1 -> Switch2/3
  Constant6/1 -> Switch3/1
  Constant7/1 -> Switch3/3
  Constant8/1 -> Switch4/1
  Constant9/1 -> Switch4/3
  Constant10/1 -> Switch5/1
  Constant11/1 -> Switch5/3
  Constant12/1 -> Switch6/1
  Constant13/1 -> Switch6/3
  Constant14/1 -> Switch7/1
  Constant15/1 -> Switch7/3
  p3/1 -> Switch1/2, Switch2/2, Switch3/2, Switch4/2, Switch6/2, Switch7/2, Switch8/2, Switch9/2, Switch5/2
  Mux/1 -> Sum of Elements/1
  Sum of Elements/1 -> Multiport Switch/1
  Constant1/1 -> Mux/1
  Switch1/1 -> Mux/2
  Switch2/1 -> Mux/3
  Switch3/1 -> Mux/4
  Switch4/1 -> Mux/5
  Switch5/1 -> Mux/6
  Switch6/1 -> Mux/7
  Switch7/1 -> Mux/8
  Switch8/1 -> Mux/9
  Switch9/1 -> Mux/10
  Constant16/1 -> Switch8/1
  Constant17/1 -> Switch8/3
  Constant18/1 -> Switch9/1
  Constant19/1 -> Switch9/3
  Multiport Switch/1 -> Product/1, Product1/1
  Constant20/1 -> Multiport Switch/2
  Constant21/1 -> Multiport Switch/3
  Constant22/1 -> Multiport Switch/4
  Constant23/1 -> Multiport Switch/5
  Constant24/1 -> Multiport Switch/6
  Constant25/1 -> Multiport Switch/7
  Constant26/1 -> Multiport Switch/8
  Constant27/1 -> Multiport Switch/9
  Constant28/1 -> Multiport Switch/10
  Constant29/1 -> Multiport Switch/11
  bililiuliangfa18_1/1 -> Product/2
  bililiuliangfa18_3/1 -> Product1/2
  Product/1 -> fa18_1/1
  Product1/1 -> fa18_3/1

== system junyakaiguangai5/Subsystem2/shoudong/Subsystem1/Signal Builder ==
  Demux : Demux  Tag=STV Demux  Outputs=1
  FromWs : FromWorkspace  Tag=STV FromWs  VariableName=tuvar  SampleTime=0  SigBuilderData=DataTag0  VnvData=DataTag1
      SigBuilderData=|
      | common.afterFinalStr = 'Extrapolate'
      | common.sampleTime = 0
      | dataSet.timeRange = [0 10]
      | dataSet.name = 'Group 1'
      | sbobj.Groups.Name = 'Group 1'
      | sbobj.Groups.Signals.Name = 'Signal 1'
      | sbobj.Groups.Signals.XData = [0 4 4 6 6 10]
      | sbobj.Groups.Signals.YData = [0 0 1 1 0 0]
  Signal 1 : Outport  Tag=STV Outport
  wires:
  Demux/1 -> Signal 1/1
  FromWs/1 -> Demux/1

== system junyakaiguangai5/Subsystem2/shoudong/Subsystem1/Signal Builder1 ==
  Demux : Demux  Tag=STV Demux  Outputs=1
  FromWs : FromWorkspace  Tag=STV FromWs  VariableName=tuvar  SampleTime=0  SigBuilderData=DataTag2  VnvData=DataTag3
      SigBuilderData=|
      | common.afterFinalStr = 'Extrapolate'
      | common.sampleTime = 0
      | dataSet.timeRange = [0 10]
      | dataSet.name = 'Group 1'
      | sbobj.Groups.Name = 'Group 1'
      | sbobj.Groups.Signals.Name = 'Signal 1'
      | sbobj.Groups.Signals.XData = [0 4 4 6 6 10]
      | sbobj.Groups.Signals.YData = [0 0 1 1 0 0]
  Signal 1 : Outport  Tag=STV Outport
  wires:
  FromWs/1 -> Demux/1
  Demux/1 -> Signal 1/1

== system junyakaiguangai5/Subsystem2/shoudong/Subsystem2/Signal Builder ==
  Demux : Demux  Tag=STV Demux  Outputs=1
  FromWs : FromWorkspace  Tag=STV FromWs  VariableName=tuvar  SampleTime=0  SigBuilderData=DataTag4  VnvData=DataTag5
      SigBuilderData=|
      | common.afterFinalStr = 'Extrapolate'
      | common.sampleTime = 0
      | dataSet.timeRange = [0 10]
      | dataSet.name = 'Group 1'
      | sbobj.Groups.Name = 'Group 1'
      | sbobj.Groups.Signals.Name = 'Signal 1'
      | sbobj.Groups.Signals.XData = [0 4 4 6 6 10]
      | sbobj.Groups.Signals.YData = [0 0 1 1 0 0]
  Signal 1 : Outport  Tag=STV Outport
  wires:
  FromWs/1 -> Demux/1
  Demux/1 -> Signal 1/1

== system junyakaiguangai5/Subsystem2/shoudong/Subsystem2/Signal Builder1 ==
  Demux : Demux  Tag=STV Demux  Outputs=1
  FromWs : FromWorkspace  Tag=STV FromWs  VariableName=tuvar  SampleTime=0  SigBuilderData=DataTag6  VnvData=DataTag7
      SigBuilderData=|
      | common.afterFinalStr = 'Extrapolate'
      | common.sampleTime = 0
      | dataSet.timeRange = [0 10]
      | dataSet.name = 'Group 1'
      | sbobj.Groups.Name = 'Group 1'
      | sbobj.Groups.Signals.Name = 'Signal 1'
      | sbobj.Groups.Signals.XData = [0 4 4 6 6 10]
      | sbobj.Groups.Signals.YData = [0 0 1 1 0 0]
  Signal 1 : Outport  Tag=STV Outport
  wires:
  Demux/1 -> Signal 1/1
  FromWs/1 -> Demux/1

== system junyakaiguangai5/Subsystem2/shoudong/Subsystem2/Signal Builder2 ==
  Demux : Demux  Tag=STV Demux  Outputs=1
  FromWs : FromWorkspace  Tag=STV FromWs  VariableName=tuvar  SampleTime=0  SigBuilderData=DataTag8  VnvData=DataTag9
      SigBuilderData=|
      | common.afterFinalStr = 'Extrapolate'
      | common.sampleTime = 0
      | dataSet.timeRange = [0 10]
      | dataSet.name = 'Group 1'
      | sbobj.Groups.Name = 'Group 1'
      | sbobj.Groups.Signals.Name = 'Signal 1'
      | sbobj.Groups.Signals.XData = [0 4 4 6 6 10]
      | sbobj.Groups.Signals.YData = [0 0 1 1 0 0]
  Signal 1 : Outport  Tag=STV Outport
  wires:
  Demux/1 -> Signal 1/1
  FromWs/1 -> Demux/1

== system junyakaiguangai5/Subsystem2/shoudong/Subsystem2/Signal Builder3 ==
  Demux : Demux  Tag=STV Demux  Outputs=1
  FromWs : FromWorkspace  Tag=STV FromWs  VariableName=tuvar  SampleTime=0  SigBuilderData=DataTag10  VnvData=DataTag11
      SigBuilderData=|
      | common.afterFinalStr = 'Extrapolate'
      | common.sampleTime = 0
      | dataSet.timeRange = [0 10]
      | dataSet.name = 'Group 1'
      | sbobj.Groups.Name = 'Group 1'
      | sbobj.Groups.Signals.Name = 'Signal 1'
      | sbobj.Groups.Signals.XData = [0 4 4 6 6 10]
      | sbobj.Groups.Signals.YData = [0 0 1 1 0 0]
  Signal 1 : Outport  Tag=STV Outport
  wires:
  FromWs/1 -> Demux/1
  Demux/1 -> Signal 1/1

== system junyakaiguangai5/Subsystem2/zidong/Subsystem/Signal Builder ==
  Demux : Demux  Tag=STV Demux  Outputs=1
  FromWs : FromWorkspace  Tag=STV FromWs  VariableName=tuvar  SampleTime=0  SigBuilderData=DataTag12  VnvData=DataTag13
      SigBuilderData=|
      | common.afterFinalStr = 'Extrapolate'
      | common.sampleTime = 0
      | dataSet.timeRange = [0 10]
      | dataSet.name = 'Group 1'
      | sbobj.Groups.Name = 'Group 1'
      | sbobj.Groups.Signals.Name = 'Signal 1'
      | sbobj.Groups.Signals.XData = [0 4 4 6 6 10]
      | sbobj.Groups.Signals.YData = [0 0 1 1 0 0]
  Signal 1 : Outport  Tag=STV Outport
  wires:
  Demux/1 -> Signal 1/1
  FromWs/1 -> Demux/1

== system junyakaiguangai5/Subsystem2/zidong/Subsystem/Signal Builder1 ==
  Demux : Demux  Tag=STV Demux  Outputs=1
  FromWs : FromWorkspace  Tag=STV FromWs  VariableName=tuvar  SampleTime=0  SigBuilderData=DataTag14  VnvData=DataTag15
      SigBuilderData=|
      | common.afterFinalStr = 'Extrapolate'
      | common.sampleTime = 0
      | dataSet.timeRange = [0 10]
      | dataSet.name = 'Group 1'
      | sbobj.Groups.Name = 'Group 1'
      | sbobj.Groups.Signals.Name = 'Signal 1'
      | sbobj.Groups.Signals.XData = [0 4 4 6 6 10]
      | sbobj.Groups.Signals.YData = [0 0 1 1 0 0]
  Signal 1 : Outport  Tag=STV Outport
  wires:
  FromWs/1 -> Demux/1
  Demux/1 -> Signal 1/1

== system junyakaiguangai5/Subsystem2/zidong/Subsystem1/Signal Builder ==
  Demux : Demux  Tag=STV Demux  Outputs=1
  FromWs : FromWorkspace  Tag=STV FromWs  VariableName=tuvar  SampleTime=0  SigBuilderData=DataTag16  VnvData=DataTag17
      SigBuilderData=|
      | common.afterFinalStr = 'Extrapolate'
      | common.sampleTime = 0
      | dataSet.timeRange = [0 10]
      | dataSet.name = 'Group 1'
      | sbobj.Groups.Name = 'Group 1'
      | sbobj.Groups.Signals.Name = 'Signal 1'
      | sbobj.Groups.Signals.XData = [0 4 4 6 6 10]
      | sbobj.Groups.Signals.YData = [0 0 1 1 0 0]
  Signal 1 : Outport  Tag=STV Outport
  wires:
  FromWs/1 -> Demux/1
  Demux/1 -> Signal 1/1

== system junyakaiguangai5/Subsystem2/zidong/Subsystem1/Signal Builder1 ==
  Demux : Demux  Tag=STV Demux  Outputs=1
  FromWs : FromWorkspace  Tag=STV FromWs  VariableName=tuvar  SampleTime=0  SigBuilderData=DataTag18  VnvData=DataTag19
      SigBuilderData=|
      | common.afterFinalStr = 'Extrapolate'
      | common.sampleTime = 0
      | dataSet.timeRange = [0 10]
      | dataSet.name = 'Group 1'
      | sbobj.Groups.Name = 'Group 1'
      | sbobj.Groups.Signals.Name = 'Signal 1'
      | sbobj.Groups.Signals.XData = [0 4 4 6 6 10]
      | sbobj.Groups.Signals.YData = [0 0 1 1 0 0]
  Signal 1 : Outport  Tag=STV Outport
  wires:
  Demux/1 -> Signal 1/1
  FromWs/1 -> Demux/1

== system junyakaiguangai5/Subsystem2/zidong/Subsystem1/Signal Builder2 ==
  Demux : Demux  Tag=STV Demux  Outputs=1
  FromWs : FromWorkspace  Tag=STV FromWs  VariableName=tuvar  SampleTime=0  SigBuilderData=DataTag20  VnvData=DataTag21
      SigBuilderData=|
      | common.afterFinalStr = 'Extrapolate'
      | common.sampleTime = 0
      | dataSet.timeRange = [0 10]
      | dataSet.name = 'Group 1'
      | sbobj.Groups.Name = 'Group 1'
      | sbobj.Groups.Signals.Name = 'Signal 1'
      | sbobj.Groups.Signals.XData = [0 4 4 6 6 10]
      | sbobj.Groups.Signals.YData = [0 0 1 1 0 0]
  Signal 1 : Outport  Tag=STV Outport
  wires:
  Demux/1 -> Signal 1/1
  FromWs/1 -> Demux/1

== system junyakaiguangai5/Subsystem2/zidong/Subsystem1/Signal Builder3 ==
  Demux : Demux  Tag=STV Demux  Outputs=1
  FromWs : FromWorkspace  Tag=STV FromWs  VariableName=tuvar  SampleTime=0  SigBuilderData=DataTag22  VnvData=DataTag23
      SigBuilderData=|
      | common.afterFinalStr = 'Extrapolate'
      | common.sampleTime = 0
      | dataSet.timeRange = [0 10]
      | dataSet.name = 'Group 1'
      | sbobj.Groups.Name = 'Group 1'
      | sbobj.Groups.Signals.Name = 'Signal 1'
      | sbobj.Groups.Signals.XData = [0 4 4 6 6 10]
      | sbobj.Groups.Signals.YData = [0 0 1 1 0 0]
  Signal 1 : Outport  Tag=STV Outport
  wires:
  FromWs/1 -> Demux/1
  Demux/1 -> Signal 1/1

== stateflow chart Subsystem2/zidong/Chart ==
  state zidong
    state SXQxieya
      state off1
        entry:
        diancifa11_1=0;
        bililiuliangfa18_3=0;
        bililiuliangfa18_4=0;
      state on1
        entry:
        diancifa11_5=1;
      state xieya1
        entry:
        bililiuliangfa18_1=1;
        bililiuliangfa18_2=1;
        p0_2=p0sheding;
      state xieya1_2
        entry:
        bililiuliangfa18_1=1;
        bililiuliangfa18_2=0;
      state xieya1_1
        entry:
        bililiuliangfa18_1=1;
        bililiuliangfa18_2=1;
      state xieya1_3
        entry:
        bililiuliangfa18_1=0;
        bililiuliangfa18_2=1;
      state xieya2
        entry:
        bililiuliangfa18_1=1;
        bililiuliangfa18_2=1;
        p0_2=p0_2-0.03;
      state xieya7_2
        entry:
        bililiuliangfa18_1=1;
        bililiuliangfa18_2=0;
      state xieya7_1
        entry:
        bililiuliangfa18_1=1;
        bililiuliangfa18_2=1;
      state xieya7_3
        entry:
        bililiuliangfa18_1=0;
        bililiuliangfa18_2=1;
      state off2
        entry:
        diancifa11_5=0;
        bililiuliangfa18_1=0;
        bililiuliangfa18_2=0;
        SXQxieyawancheng=1;
      state xieya8
        entry:
        diancifa11_5=1;
        bililiuliangfa18_1=1;
        bililiuliangfa18_2=1;
      (default) -> zidong.SXQxieya.off1
      zidong.SXQxieya.off1 -> zidong.SXQxieya.on1
      zidong.SXQxieya.on1 -> xieya1 : after(500,tick)
      xieya1 -> (junction 96)
      (junction 96) -> xieya1_2 [order 2] : [p2<=p0_2&&p3>p0_2]
      (junction 96) -> xieya1_1 [order 1] : [p2>p0_2&&p3>p0_2]
      xieya1_2 -> (junction 96)
      xieya1_3 -> (junction 96)
      xieya1_1 -> (junction 96)
      (junction 96) -> xieya1_3 [order 3] : [p2>p0_2&&p3<=p0_2]
      (junction 96) -> xieya2 [order 4] : [p2<=p0_2&&p3<=p0_2]
      (junction 97) -> (junction 96) [order 2] : [p0_2>p0_0]
      xieya2 -> (junction 97)
      (junction 97) -> (junction 98) [order 1] : [p0_2<=p0_0]
      (junction 98) -> xieya7_2 [order 2] : [p2<=p0_0&&p3>p0_0]
      xieya7_2 -> (junction 98)
      (junction 98) -> xieya7_1 [order 1] : [p2>p0_0&&p3>p0_0]
      xieya7_3 -> (junction 98)
      (junction 98) -> xieya7_3 [order 3] : [p2>p0_0&&p3<=p0_0]
      xieya7_1 -> (junction 98)
      (junction 98) -> xieya8 [order 4] : [p2<=p0_0&&p3<=p0_0]
      (junction 99) -> (junction 98) [order 2] : [p2>p0_0||p3>p0_0]
      (junction 99) -> zidong.SXQxieya.off2 [order 1] : [p2<=p0_0&&p3<=p0_0]
      xieya8 -> (junction 99) : after(3000,tick)
    state kaiguangai
      state start
        entry:
        xuansong=0;
        xuanjin=0;
        suoding=0;
        jiesuo=0;
        kaigaikaishi=0;
        guangaikaishi=0;
        diancifa20=0;
      state on5
        entry:
        jiesuo=1;
      state off5
        entry:
        jiesuo=0;
      state on1
        entry:diancifa20=1;
      state on6
        entry:
        guangaikaishi=1;
      state on2
        entry:
        xuansong=1;
      state on7
        entry:
        guangaikaishi=0;
        diancifa20=1;
      state off1
        entry:
        xuansong=0;
      state on8
        entry:
        xuanjin=1;
      state off2
        entry:
        diancifa20=0;
        SQshiyabuchangwancheng=1;
      state off6
        entry:
        xuanjin=0;
      state on3
        entry:
        kaigaikaishi=1;
      state on4
        entry:
        kaigaikaishi=0;
        suoding=1;
      state off7
        entry:
        diancifa20=0;
        SQxuanjinjianyawancheng=1;
        guangaiwancheng=1;
      state off3
        entry:
        suoding=0;
      state off4
        entry:
        kaigaiwancheng=1;
      (default) -> zidong.kaiguangai.start
      zidong.kaiguangai.off4 -> on5 : after(5000,tick)
      on5 -> zidong.kaiguangai.off5 : [jiesuodaowei1==1&&jiesuodaowei2==1]
      zidong.kaiguangai.start -> zidong.kaiguangai.on1
      zidong.kaiguangai.off5 -> on6 : after(1000,tick)
      zidong.kaiguangai.on1 -> zidong.kaiguangai.on2 : [liuliangji==1&&p1==p2]
      on6 -> on7 : [guangaijieshu==1]
      zidong.kaiguangai.on2 -> zidong.kaiguangai.off1 : [xuansongdaowei1==1&&xuansongdaowei2==1]
      on7 -> on8 : [liuliangji==1&&p1==p2]
      zidong.kaiguangai.off1 -> zidong.kaiguangai.off2 : after(500,tick)
      on8 -> zidong.kaiguangai.off6 : [xuanjindaowei1==1&&xuanjindaowei2==1]
      zidong.kaiguangai.off2 -> zidong.kaiguangai.on3 : after(1000,tick)
      zidong.kaiguangai.off6 -> off7 : after(500,tick)
      zidong.kaiguangai.on3 -> on4 : [kaigaijieshu==1]
      on4 -> zidong.kaiguangai.off3 : [suodingdaowei1==1&&suodingdaowei2==1]
      zidong.kaiguangai.off3 -> zidong.kaiguangai.off4 : after(500,tick)
    state SCjiaya
      state off1
        entry:diancifa11_1=0;
        diancifa11_2=0;
        diancifa16_1=0;
      state on1
        entry:diancifa11_1=1;
        diancifa11_2=1;
        diancifa16_1=0;
      state off2
        entry:
        diancifa11_1=0;
        diancifa11_2=0;
        diancifa16_1=0;
      state on3
        entry:diancifa11_1=1;
        diancifa11_2=1;
        diancifa16_1=0;
      state on2
        entry:diancifa16_1=1;
      state off3
        entry:
        diancifa11_1=0;
        diancifa11_2=0;
        diancifa16_1=0;
      state off4
        entry:
        SCjiayawancheng=1;
      (default) -> zidong.SCjiaya.off1
      zidong.SCjiaya.off1 -> zidong.SCjiaya.on1
      zidong.SCjiaya.on1 -> zidong.SCjiaya.off2 : [p1>=p1sheding-0.005]
      zidong.SCjiaya.off2 -> (junction 140) : after(5000,tick)
      zidong.SCjiaya.on2 -> (junction 140)
      zidong.SCjiaya.on3 -> (junction 140)
      (junction 140) -> zidong.SCjiaya.on2 [order 2] : [p1>p1sheding+0.005]
      (junction 140) -> zidong.SCjiaya.on3 [order 1] : [p1<(p1sheding-0.005)]
      (junction 140) -> zidong.SCjiaya.off3 [order 3] : [p1>=(p1sheding-0.005)&&p1<=p1sheding+0.005]
      zidong.SCjiaya.off3 -> zidong.SCjiaya.off4
    state SCzhushui
      state off4
        entry:diancifa16_1=0;
        diancifa3=0;
      state on2
        entry:diancifa16_1=1;
      state on3
        entry:diancifa3=1;
      state off1
        entry:diancifa3=0;
      state off2
        entry:diancifa16_1=0;
      state off3
        entry:
        SCzhushuiwancheng=1;
      (default) -> zidong.SCzhushui.off4
      zidong.SCzhushui.off4 -> zidong.SCzhushui.on2 : [SCzhushui==1]
      zidong.SCzhushui.on2 -> zidong.SCzhushui.on3 : after(20,tick)
      zidong.SCzhushui.on3 -> zidong.SCzhushui.off1 : [fuqiuyeweikongzhiqi==1]
      zidong.SCzhushui.off1 -> zidong.SCzhushui.off2
      zidong.SCzhushui.off2 -> zidong.SCzhushui.off3
    state SXQjunya
      state jiaya1_1
        entry:
        bililiuliangfa18_3=1;
        bililiuliangfa18_4=1;
      state jiaya7_1
        entry:
        bililiuliangfa18_3=1;
        bililiuliangfa18_4=1;
      state jiaya2
        entry:
        bililiuliangfa18_3=1;
        bililiuliangfa18_4=1;
        p0_1=p0_1+0.03;
      state off1
        entry:
        diancifa20=0;
        bililiuliangfa18_1=0;
        bililiuliangfa18_2=0;
      state jiaya1
        entry:
        bililiuliangfa18_3=1;
        bililiuliangfa18_4=1;
        p0_1=p0_0;
      state on1
        entry:
        diancifa11_1=1;
        diancifa11_5=1;
      state off2
        entry:
        diancifa11_5=0;
        bililiuliangfa18_3=0;
        bililiuliangfa18_4=0;
      state jiance1_35
        entry:
        bililiuliangfa18_1=0;
        bililiuliangfa18_2=1;
      state jiance1_34
        entry:
        bililiuliangfa18_1=1;
        bililiuliangfa18_2=0;
      state jiaya7_3
        entry:
        bililiuliangfa18_3=0;
        bililiuliangfa18_4=1;
      state jiaya7_2
        entry:
        bililiuliangfa18_3=1;
        bililiuliangfa18_4=0;
      state jiaya1_2
        entry:
        bililiuliangfa18_3=1;
        bililiuliangfa18_4=0;
      state jiaya1_3
        entry:
        bililiuliangfa18_3=0;
        bililiuliangfa18_4=1;
      state jiance1_33
        entry:
        diancifa11_5=0;
      state jiance2_34
        entry:
        bililiuliangfa18_3=1;
        bililiuliangfa18_4=0;
      state jiance2_33
        entry:
        diancifa11_5=0;
      state jiance2_32
        entry:
        bililiuliangfa18_3=1;
        bililiuliangfa18_4=1;
      state jiance2_31
        entry:
        diancifa11_5=1;
      state jiance1_36
        entry:
        diancifa11_5=0;
        bililiuliangfa18_1=0;
        bililiuliangfa18_2=0;
      state jiance1_32
        entry:
        bililiuliangfa18_1=1;
        bililiuliangfa18_2=1;
      state jiance2_35
        entry:
        bililiuliangfa18_3=0;
        bililiuliangfa18_4=1;
      state off5
        entry:
        diancifa11_5=0;
        bililiuliangfa18_3=0;
        bililiuliangfa18_4=0;
      state jiance2_36
        entry:
        diancifa11_5=0;
        bililiuliangfa18_3=0;
        bililiuliangfa18_4=0;
      state jiance1_31
        entry:
        diancifa11_5=1;
      state off3
        entry:
        diancifa11_5=0;
        bililiuliangfa18_3=0;
        bililiuliangfa18_4=0;
      state off6
        entry:
        diancifa11_1=0;
        SXQjunyawancheng=1;
      state jiance1_21
        entry:
        bililiuliangfa18_1=1;
      state off4
        entry:
        diancifa11_5=0;
        bililiuliangfa18_3=0;
        bililiuliangfa18_4=0;
      state jiance1_22
        entry:
        bililiuliangfa18_1=0;
      state jiance1_11
        entry:
        diancifa11_5=1;
      state jiance1_14
        entry:
        bililiuliangfa18_2=0;
      state jiance2_11
        entry:
        diancifa11_5=1;
      state jiance2_14
        entry:
        bililiuliangfa18_4=0;
      state jiance2_21
        entry:
        bililiuliangfa18_3=1;
      state jiance1_12
        entry:
        bililiuliangfa18_2=1;
      state jiance1_13
        entry:
        diancifa11_5=0;
      state jiance2_22
        entry:
        bililiuliangfa18_3=0;
      state jiance2_12
        entry:
        bililiuliangfa18_4=1;
      state jiance2_13
        entry:
        diancifa11_5=0;
      jiaya1_1 -> (junction 157)
      (junction 157) -> jiaya2 [order 4] : [p2>=p0_1&&p3>=p0_1]
      (junction 157) -> jiaya1_1 [order 1] : [p2<p0_1&&p3<p0_1]
      jiaya7_1 -> (junction 159)
      (junction 159) -> jiaya7_1 [order 1] : [p2<p0sheding&&p3<p0sheding]
      (default) -> zidong.SXQjunya.off1
      jiaya2 -> (junction 158)
      (junction 159) -> zidong.SXQjunya.off2 [order 4] : [p2>=p0sheding&&p3>=p0sheding]
      jiaya1 -> (junction 157)
      (junction 158) -> (junction 157) [order 2] : [p0_1<p0sheding]
      (junction 158) -> (junction 159) [order 1] : [p0_1>=p0sheding]
      (junction 157) -> jiaya1_3 [order 3] : [p2<p0_1&&p3>=p0_1]
      zidong.SXQjunya.on1 -> jiaya1 : after(500,tick)
      zidong.SXQjunya.off1 -> zidong.SXQjunya.on1
      jiaya1_3 -> (junction 157)
      (junction 159) -> jiaya7_2 [order 2] : [p2>=p0sheding&&p3<p0sheding]
      (junction 159) -> jiaya7_3 [order 3] : [p2<p0sheding&&p3>=p0sheding]
      jiaya7_3 -> (junction 159)
      jiaya7_2 -> (junction 159)
      (junction 157) -> jiaya1_2 [order 2] : [p2>=p0_1&&p3<p0_1]
      jiaya1_2 -> (junction 157)
      jiance1_35 -> (junction 160)
      zidong.SXQjunya.off2 -> (junction 163) : after(3000,tick)
      jiance1_34 -> (junction 160)
      (junction 160) -> jiance1_35 [order 2] : [p2>(p0sheding+0.012)&&p3<=(p0sheding+0.012)]
      jiance1_33 -> jiance1_34
      jiance2_33 -> jiance2_34
      (junction 160) -> jiance1_33 [order 1] : [p2<=(p0sheding+0.012)&&p3>(p0sheding+0.012)]
      (junction 160) -> jiance1_36 [order 3] : [p2<=(p0sheding+0.012)&&p3<=(p0sheding+0.012)]
      jiance1_32 -> (junction 160)
      jiance2_32 -> (junction 161)
      (junction 161) -> jiance2_33 [order 1] : [p2>=(p0sheding-0.01)&&p3<(p0sheding-0.001)]
      jiance2_34 -> (junction 161)
      jiance2_31 -> jiance2_32
      (junction 161) -> jiance2_35 [order 2] : [p2<(p0sheding-0.01)&&p3>=(p0sheding-0.001)]
      jiance2_35 -> (junction 161)
      (junction 161) -> jiance2_36 [order 3] : [p2>=(p0sheding-0.01)&&p3>=(p0sheding-0.001)]
      (junction 165) -> jiance2_31 [order 5] : [p2<(p0sheding-0.01)&&p3<(p0sheding-0.001)]
      jiance1_31 -> jiance1_32
      jiance1_36 -> (junction 163)
      (junction 163) -> jiance1_31 [order 3] : [p2>(p0sheding+0.012)&&p3>(p0sheding+0.012)]
      (junction 165) -> zidong.SXQjunya.off5 [order 1] : [p2>=(p0sheding-0.01)&&p2<=(p0sheding+0.012)&&p3>=(p0sheding-0.01)&&p3<=(p0sheding+0.012)]
      zidong.SXQjunya.off3 -> (junction 162) : after(1000,tick)
      (junction 162) -> (junction 165) [order 1] : [p2<=(p0sheding+0.012)&&p3<=(p0sheding+0.012)]
      (junction 163) -> zidong.SXQjunya.off3 [order 4] : [p2<=(p0sheding+0.012)&&p3<=(p0sheding+0.012)]
      (junction 162) -> (junction 163) [order 2] : [p2>(p0sheding+0.012)||p3>(p0sheding+0.012)]
      zidong.SXQjunya.off5 -> (junction 164) : after(1000,tick)
      jiance2_36 -> (junction 165)
      (junction 163) -> jiance1_21 [order 2] : [p2<=(p0sheding+0.012)&&p3>(p0sheding+0.012)]
      (junction 166) -> (junction 165) [order 2] : [p2<=(p0sheding+0.012)&&p3<=(p0sheding+0.012)]
      (junction 166) -> (junction 163) [order 1] : [p2>(p0sheding+0.012)||p3>(p0sheding+0.012)]
      jiance1_22 -> (junction 163)
      jiance1_14 -> (junction 163)
      (junction 163) -> jiance1_11 [order 1] : [p2>(p0sheding+0.012)&&p3<=(p0sheding+0.012)]
      (junction 164) -> (junction 165) [order 2] : [p2<(p0sheding-0.01)||p2>(p0sheding+0.012)||p3<(p0sheding-0.01)||p3>(p0sheding+0.012)]
      (junction 164) -> zidong.SXQjunya.off6 [order 1] : [p2>=(p0sheding-0.01)&&p2<=(p0sheding+0.012)&&p3>=(p0sheding-0.01)&&p3<=(p0sheding+0.012)]
      (junction 165) -> zidong.SXQjunya.off4 [order 2] : [p2>(p0sheding+0.012)||p3>(p0sheding+0.012)]
      (junction 165) -> jiance2_21 [order 4] : [p2>=(p0sheding-0.01)&&p3<(p0sheding-0.001)]
      jiance2_14 -> (junction 165)
      jiance2_22 -> (junction 165)
      (junction 165) -> jiance2_11 [order 3] : [p2<(p0sheding-0.01)&&p3>=(p0sheding-0.001)]
      jiance1_21 -> jiance1_22 : [p2<=(p0sheding+0.012)&&p3<=(p0sheding+0.012)]
      zidong.SXQjunya.off4 -> (junction 166) : after(1000,tick)
      jiance1_11 -> jiance1_12
      jiance1_13 -> jiance1_14
      jiance2_11 -> jiance2_12
      jiance2_13 -> jiance2_14
      jiance2_21 -> jiance2_22 : [p2>=(p0sheding-0.01)&&p3>=(p0sheding-0.001)]
      jiance1_12 -> jiance1_13 : [p2<=(p0sheding+0.012)&&p3<=(p0sheding+0.012)]
      jiance2_12 -> jiance2_13 : [p2>=(p0sheding-0.01)&&p3>=(p0sheding-0.001)]
    (default) -> SCzhushui
    zidong.SCzhushui.off3 -> SCjiaya : after(5000,tick)
    off7 -> SXQxieya : after(5000,tick)
    zidong.SCjiaya.off4 -> SXQjunya : after(5000,tick)
    zidong.SXQjunya.off6 -> kaiguangai : after(5000,tick)
  state start
    en:
    diancifa11_1=0;
    diancifa11_2=0;
    diancifa11_5=0;
    diancifa20=0
    diancifa16_1=0;
    diancifa3=0;
    diancifa21=0;
    bililiuliangfa18_1=0;
    bililiuliangfa18_2=0;
    bililiuliangfa18_3=0;
    bililiuliangfa18_4=0;
    xuansong=0;
    xuanjin=0;
    suoding=0;
    jiesuo=0;
    kaigaikaishi=0;
    guangaikaishi=0;
  state off111
    en:
    diancifa11_1=0;
    diancifa11_2=0;
    diancifa11_5=0;
    diancifa20=0
    diancifa16_1=0;
    diancifa3=0;
    diancifa21=0;
    bililiuliangfa18_1=0;
    bililiuliangfa18_2=0;
    bililiuliangfa18_3=0;
    bililiuliangfa18_4=0;
    xuansong=0;
    xuanjin=0;
    suoding=0;
    jiesuo=0;
    SCzhushuiwancheng=0;
    SCjiayawancheng=0;
    SXQjunyawancheng=0;
    SQshiyabuchangwancheng=0;
    kaigaikaishi=0;
    kaigaiwancheng=0;
    SQxuanjinjianyawancheng=0;
    guangaikaishi=0;
    guangaiwancheng=0;
    SXQxieyawancheng=0;
  (default) -> start
  start -> zidong : [start==1]
  zidong -> off111 : [jieshu==1]
  data: start input double; diancifa11_1 output double; diancifa11_2 output double; diancifa11_5 output double; SCzhushui input double; fuqiuyeweikongzhiqi input double; diancifa20 output double; diancifa16_1 output double; diancifa3 output double; SCjiaya input double; SXQjunya input double; diancifa21 output double; suoding output double; jiesuo output double; xuansong output double; xuanjin output double; bililiuliangfa18_1 output double; bililiuliangfa18_2 output double; bililiuliangfa18_3 output double; bililiuliangfa18_4 output double; SXQxieya input double; p1 input double; p1sheding input double; liuliangji input double; p2 input double; p3 input double; p0_0 input double; p0sheding input double; kaigaikaishi output double; guangaikaishi output double; SCzhushuiwancheng output double; SCjiayawancheng output double; SXQjunyawancheng output double; SXQxieyawancheng output double; SQshiyabuchangwancheng output double; SQxuanjinjianyawancheng output double; kaigaiwancheng output double; guangaiwancheng output double; xuansongdaowei1 input double; xuansongdaowei2 input double; xuanjindaowei1 input double; xuanjindaowei2 input double; suodingdaowei1 input double; suodingdaowei2 input double; jiesuodaowei1 input double; jiesuodaowei2 input double; kaigaijieshu input double; guangaijieshu input double; p0_1 local double; p0_2 local double; jieshu input double; zidongkaigai input double; zidongguangai input double
